simulink model "controlNoLineal"  (R2023b)
settings: Solver=VariableStepAuto  StartTime=0.0  StopTime=10.0  RelTol=1e-3
settings Model: Creator=nmestanza  LastModifiedBy=nmestanza

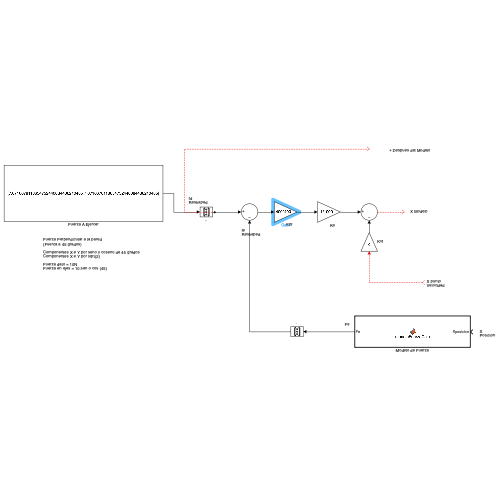
[thumbnail: Simulink's stored preview of the top-level diagram]
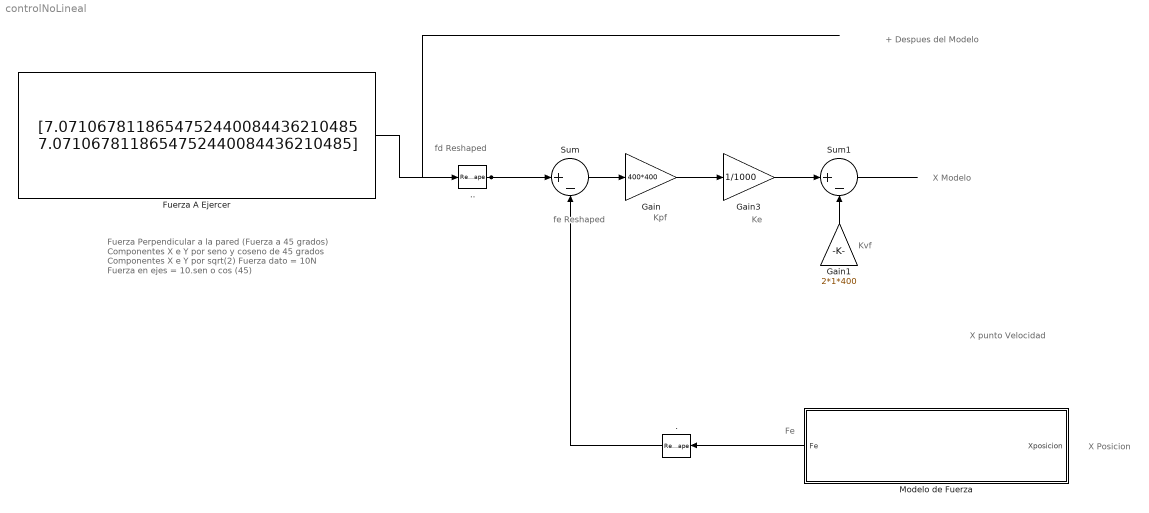
== system controlNoLineal ==
  note: X Modelo
  note: + Despues del Modelo
  note: X
      | Posicion
  note: X punto
      | Velocidad
  note: Fe
  note: fe
      | Reshaped
  note: Kvf
  note: Kpf
  note: Fuerza Perpendicular a la pared
      | (Fuerza a 45 grados)
      |
      | Componentes X e Y por seno y coseno de 45 grados
      | Componentes X e Y por sqrt(2)
      |
      | Fuerza dato = 10N
      | Fuerza en ejes = 10.sen o cos (45)
  note: Ke
  note: fd
      | Reshaped
  . : Reshape  OutputDimensionality=Column vector (2-D)
  .. : Reshape  OutputDimensionality=Column vector (2-D)
  Fuerza A Ejercer : Constant  Value=[7.0710678118654752440084436210485 7.0710678118654752440084436210485]
  Gain : Gain  Gain=400*400
  Gain1 : Gain  Gain=2*1*400
  Gain3 : Gain  Gain=1/1000
  Modelo de Fuerza : MATLAB Function  TreatAsAtomicUnit=on
  Sum : Sum  Inputs=|+-
  Sum1 : Sum  Inputs=|+-
  wires:
  Modelo de Fuerza/1(Fe) -> ./1
  Fuerza A Ejercer/1 -> ../1
  Gain3/1 -> Sum1/1
  Gain/1 -> Gain3/1
  Sum/1 -> Gain/1
  Gain1/1 -> Sum1/2
  Sum1/1 -> ?
  ../1 -> Sum/1
  ? -> Gain1/1
  ./1 -> Sum/2

== matlab function controlNoLineal/Modelo de Fuerza ==
  data: Xposicion input; Fe output
%Input: Vector de coordenadas bidimensionales Xposicion como entrada
%Output: Vector de fuerzas bidimensionales Fe 

%Description: Evalar la posición del punto representado por las coordenadas 
%Xposicion con respecto a la pared 
%En base a ello, calcula la fuerza correspondiente.

function Fe = modeloFuerzaCalc(Xposicion)

kEnv = 1000; %N/mm
ejeY = Xposicion(2);
ejeX = Xposicion(1);

%Pared interseca el plano XY en una línea que contiene los puntos (2; 0) y (0; 2)
%Verification Total:
%limY = (ejeX*(-1)+2)/1 = 2 - ejeX
%limX = ((ejeY*1)-2)/-1 = 2 - ejeY
%Por ende:
%ejeX < limX y ejeY< limY
%ejeY < 2 - ejeX ; ejeX < 2 - ejeY
%ejeY + ejeX - 2 + ejeX + ejeY  -2 < 0 
%2ejeX + 2ejeY - 4 < 0 -> ejeX + ejeY - 2 < 0

%Verifico si el punto está en el lado negativo de la pared
%Calculo la distancia entre el punto y la pared
%Defino la fuerza en función de esa distancia.

if (2-ejeX-ejeY) <= 0 

    distancia = abs(2-ejeX-ejeY)/sqrt(1^2+1^2);
    Fe = [distancia*kEnv*sqrt(2)/2, distancia*kEnv*sqrt(2)/2];

%Verifico si el punto está en el lado positivo de la pared 

else 

    Fe=[0, 0];



end
